simulink model "analyze"  (R2014a)
settings: Solver=FixedStepDiscrete  StartTime=0.0  StopTime=1  FixedStep=0.02  RelTol=1e-3
InitFcn:
  | Veh_Par_wxt
values from neighbouring files (symbols this model uses):
  ag_thr = 0.4*g    (= 3.924)    [Veh_Par_wxt.m]
  B = 2.25    [Veh_Par_wxt.m]
  bra_pre_em = 12    [Veh_Par_wxt.m]
  bra_pre_gz2 = 12/3    (= 4)    [Veh_Par_wxt.m]
  bra_pre_gz34 = 12/3    (= 4)    [Veh_Par_wxt.m]
  bra_pre_yd = 12/2    (= 6)    [Veh_Par_wxt.m]
  brakepre_dem_data = [0 1 2 3 4 5 6 7 8 9 10 11 12]    [Veh_Par_wxt.m]
  brakeTrq_dem_data = [0 218.198 436.396 654.594 872.792 1090.99 1309.188 1527.386 1745.584 1963.782 2181.98 2400.178 2618.376]    [Veh_Par_wxt.m]
  bratrq_max = 4*2618.376    (= 10473.504)    [Veh_Par_wxt.m]
  eff_tran = 0.75    [Veh_Par_wxt.m]
  G = Mass*g    (= 36297)    [Veh_Par_wxt.m]
  kd1 = 1    [Veh_Par_wxt.m]
  kd2 = 1    [Veh_Par_wxt.m]
  kd3 = 1    [Veh_Par_wxt.m]
  ki1 = 1    [Veh_Par_wxt.m]
  ki2 = 1    [Veh_Par_wxt.m]
  ki3 = 1    [Veh_Par_wxt.m]
  kp1 = 1    [Veh_Par_wxt.m]
  kp2 = 1    [Veh_Par_wxt.m]
  kp3 = 1    [Veh_Par_wxt.m]
  L = 3.12    [Veh_Par_wxt.m]
  premax = 12    [Veh_Par_wxt.m]
  Radius = 0.20    (= 0.2)    [Veh_Par_wxt.m]
  s_opt_yi_add = 0.05    [Veh_Par_wxt.m]
  s_opt_zhuan_add = 0.05    [Veh_Par_wxt.m]
  spd_map_mot = [0 100 200 300 360 400 500 600 700 800 900]*tras_ratio    [Veh_Par_wxt.m]
  spdmax = 900*tras_ratio    (= 5580)    [Veh_Par_wxt.m]
  speed_thr_park = 5/3.6/Radius*30/pi    (= 66.3145596216)    [Veh_Par_wxt.m]
  tras_ratio = 6.2    [Veh_Par_wxt.m]
  trq_map_mot = [1200 1200 1200 1200 1200 1080 864 720 617 540 480]/tras_ratio    [Veh_Par_wxt.m]
  trqmax = 80    [Veh_Par_wxt.m]
  v_thr1_b = 5    [Veh_Par_wxt.m]
  v_thr2_b = 20    [Veh_Par_wxt.m]
  v_thr_park = 5    [Veh_Par_wxt.m]
undefined symbols (not defined in the file or in its folder): DiscIntNeverNeededParam
libraries: simulink x231, ec5744lib x19
(part 6 of 16)

== matlab function analyze/MainControl/mode_control/backward/backward/Drive/目标转向力矩确定模块/MATLAB Function1 ==
  data: v_act input; Rturn_min_ag output; ag_thr input
function Rturn_min_ag = fcn(v_act,ag_thr)
%#codegen

    Rturn_min_ag=(v_act/3.6)^2/ag_thr;
end

== matlab function analyze/MainControl/mode_control/backward/backward/Drive/驱动防滑控制TCS/直行TCS/直行/HeartBeat1 ==
  data: life_pre input; life output
function life = fcn(life_pre)
%#codegen
life=life_pre+1;
if life>15
    life=0;
end
end

== matlab function analyze/MainControl/mode_control/backward/backward/Drive/驱动防滑控制TCS/转向TCS/MATLAB Function ==
  data: steer_dem input; y output
function y = fcn(steer_dem)
%#codegen左转为0，右转为1
if steer_dem>0
    y=0;
else
    y = 1;
end
end

== matlab function analyze/MainControl/mode_control/backward/backward/Drive/驱动防滑控制TCS/转向TCS/右转/MATLAB Function ==
  data: s_act_lf input; flag_lf output; s_opt_zhuan input; s_opt_zhuan_add input; flag_lf_pre input
function flag_lf = fcn(s_act_lf,s_opt_zhuan,s_opt_zhuan_add,flag_lf_pre)
%#codegen
if s_act_lf>s_opt_zhuan+s_opt_zhuan_add
    flag_lf=1;
elseif s_act_lf<s_opt_zhuan
    flag_lf = 0;
else
    flag_lf=flag_lf_pre;
end
end

== matlab function analyze/MainControl/mode_control/backward/backward/Drive/驱动防滑控制TCS/转向TCS/右转/前轮滑转/HeartBeat ==
  data: life_pre input; life output
function life = fcn(life_pre)
%#codegen
life=life_pre+1;
if life>15
    life=0;
end
end

== matlab function analyze/MainControl/mode_control/backward/backward/Drive/驱动防滑控制TCS/转向TCS/左转/MATLAB Function ==
  data: s_act_lf input; flag_lf output; s_opt_zhuan input; s_opt_zhuan_add input; flag_lf_pre input
function flag_lf = fcn(s_act_lf,s_opt_zhuan,s_opt_zhuan_add,flag_lf_pre)
%#codegen
if s_act_lf>s_opt_zhuan+s_opt_zhuan_add
    flag_lf=1;
elseif s_act_lf<s_opt_zhuan
    flag_lf = 0;
else
    flag_lf=flag_lf_pre;
end
end

== matlab function analyze/MainControl/mode_control/backward/backward/Drive/驱动防滑控制TCS/转向TCS/左转/前后轮均滑转/HeartBeat1 ==
  data: life_pre input; life output
function life = fcn(life_pre)
%#codegen
life=life_pre+1;
if life>15
    life=0;
end
end

== matlab function analyze/MainControl/mode_control/backward/backward/Drive/驱动防滑控制TCS/转向TCS/左转/无滑转/HeartBeat1 ==
  data: life_pre input; life output
function life = fcn(life_pre)
%#codegen
life=life_pre+1;
if life>15
    life=0;
end
end

== matlab function analyze/InputSignalProcess/MATLAB Function4 ==
  data: mode_dem input; mode_dem1 output
function mode_dem1 = fcn(mode_dem)
%#codegen
if mode_dem==0 || mode_dem==4 || mode_dem==5 
    mode_dem1=1;
elseif mode_dem==1 || mode_dem==6 || mode_dem==7 
    mode_dem1=3
elseif mode_dem==2 || mode_dem==3
    mode_dem1=4;
else 
    mode_dem1=2;
end
end

== system analyze/Data_Input/MCU1_VCU3/MCU1_VCU3 ==
  input : Inport
  Enable : EnablePort
  Demux : Demux  Outputs=8
  M2Current_Ad : Sum
  M2Current_Convert : DataTypeConversion  OutDataTypeStr=uint32
  M2Current_F : Gain  Gain=0.5
  M2Current_L : simulink/Logic and Bit Operations/Bitwise Operator  logicop=AND  UseBitMask=on  BitMask=65520  BitMaskRealWorld=Stored Integer
  M2Current_O : Constant  Value=-600  OutDataTypeStr=single
  M2Current_S : ArithShift  BitShiftNumber=4
  M2Current_Sub : Subsystem
  M2Current_sat : Saturate  UpperLimit=1447.5  LowerLimit=-600
  M2Currentcv : DataTypeConversion
  M2Currentinput3_Ad : Sum
  M2Currentinput3_C : Constant  Value=256
  M2Currentinput3_P : Product
  M2Direction_Ad : Sum
  M2Direction_Convert : DataTypeConversion  OutDataTypeStr=uint32
  M2Direction_F : Gain
  M2Direction_L : simulink/Logic and Bit Operations/Bitwise Operator  logicop=AND  UseBitMask=on  BitMask=128  BitMaskRealWorld=Stored Integer
  M2Direction_O : Constant  Value=0  OutDataTypeStr=single
  M2Direction_S : ArithShift  BitShiftNumber=7
  M2Direction_Sub : Subsystem
  M2Direction_sat : Saturate  UpperLimit=1  LowerLimit=0
  M2Directioncv : DataTypeConversion
  M2HeartBeat_Ad : Sum
  M2HeartBeat_Convert : DataTypeConversion  OutDataTypeStr=uint32
  M2HeartBeat_F : Gain
  M2HeartBeat_L : simulink/Logic and Bit Operations/Bitwise Operator  logicop=AND  UseBitMask=on  BitMask=15  BitMaskRealWorld=Stored Integer
  M2HeartBeat_O : Constant  Value=0  OutDataTypeStr=single
  M2HeartBeat_S : ArithShift
  M2HeartBeat_Sub : Subsystem
  M2HeartBeat_sat : Saturate  UpperLimit=15  LowerLimit=0
  M2HeartBeatcv : DataTypeConversion
  M2InputVolt_Ad : Sum
  M2InputVolt_Convert : DataTypeConversion  OutDataTypeStr=uint32
  M2InputVolt_F : Gain  Gain=0.25
  M2InputVolt_L : simulink/Logic and Bit Operations/Bitwise Operator  logicop=AND  UseBitMask=on  BitMask=4095  BitMaskRealWorld=Stored Integer
  M2InputVolt_O : Constant  Value=0  OutDataTypeStr=single
  M2InputVolt_S : ArithShift
  M2InputVolt_Sub : Subsystem
  M2InputVolt_sat : Saturate  UpperLimit=1023.75  LowerLimit=0
  M2InputVoltcv : DataTypeConversion
  M2InputVoltinput8_Ad : Sum
  M2InputVoltinput8_C : Constant  Value=256
  M2InputVoltinput8_P : Product
  M2Speed_Ad : Sum
  M2Speed_Convert : DataTypeConversion  OutDataTypeStr=uint32
  M2Speed_F : Gain  Gain=5
  M2Speed_L : simulink/Logic and Bit Operations/Bitwise Operator  logicop=AND  UseBitMask=on  BitMask=65535  BitMaskRealWorld=Stored Integer
  M2Speed_O : Constant  Value=-5000  OutDataTypeStr=single
  M2Speed_S : ArithShift
  M2Speed_Sub : Subsystem
  M2Speed_sat : Saturate  UpperLimit=322675  LowerLimit=-5000
  M2Speedcv : DataTypeConversion
  M2Speedinput6_Ad : Sum
  M2Speedinput6_C : Constant  Value=256
  M2Speedinput6_P : Product
  M2State_Ad : Sum
  M2State_Convert : DataTypeConversion  OutDataTypeStr=uint32
  M2State_F : Gain
  M2State_L : simulink/Logic and Bit Operations/Bitwise Operator  logicop=AND  UseBitMask=on  BitMask=112  BitMaskRealWorld=Stored Integer
  M2State_O : Constant  Value=0  OutDataTypeStr=single
  M2State_S : ArithShift  BitShiftNumber=4
  M2State_Sub : Subsystem
  M2State_sat : Saturate  UpperLimit=7  LowerLimit=0
  M2Statecv : DataTypeConversion
  M2Torque_Ad : Sum
  M2Torque_Convert : DataTypeConversion  OutDataTypeStr=uint32
  M2Torque_F : Gain  Gain=0.25
  M2Torque_L : simulink/Logic and Bit Operations/Bitwise Operator  logicop=AND  UseBitMask=on  BitMask=4095  BitMaskRealWorld=Stored Integer
  M2Torque_O : Constant  Value=-300  OutDataTypeStr=single
  M2Torque_S : ArithShift
  M2Torque_Sub : Subsystem
  M2Torque_sat : Saturate  UpperLimit=723.75  LowerLimit=-300
  M2Torquecv : DataTypeConversion
  M2Torqueinput2_Ad : Sum
  M2Torqueinput2_C : Constant  Value=256
  M2Torqueinput2_P : Product
  M2InputVolt_Out : Outport
  M2Speed_Out : Outport  Port=2
  M2Direction_Out : Outport  Port=3
  M2State_Out : Outport  Port=4
  M2HeartBeat_Out : Outport  Port=5
  M2Current_Out : Outport  Port=6
  M2Torque_Out : Outport  Port=7
  wires:
  M2Torque_F/1 -> M2Torque_Ad/1
  M2Torque_O/1 -> M2Torque_Ad/2
  M2Torque_Ad/1 -> M2Torque_sat/1
  M2Torque_sat/1 -> M2Torque_Out/1
  Demux/2 -> M2Torqueinput2_P/1, M2Currentinput3_Ad/2
  M2Torqueinput2_C/1 -> M2Torqueinput2_P/2
  M2Torqueinput2_P/1 -> M2Torqueinput2_Ad/1
  Demux/1 -> M2Torqueinput2_Ad/2
  M2Torqueinput2_Ad/1 -> M2Torque_Sub/1(In1)
  M2Torque_Sub/1(Out1) -> M2Torque_Convert/1
  M2Torque_Convert/1 -> M2Torque_L/1
  M2Torque_L/1 -> M2Torque_S/1
  M2Torque_S/1 -> M2Torquecv/1
  M2Torquecv/1 -> M2Torque_F/1
  M2State_F/1 -> M2State_Ad/1
  M2State_O/1 -> M2State_Ad/2
  M2State_Ad/1 -> M2State_sat/1
  M2State_sat/1 -> M2State_Out/1
  Demux/4 -> M2HeartBeat_Sub/1(In1), M2Direction_Sub/1(In1), M2State_Sub/1(In1)
  M2State_Sub/1(Out1) -> M2State_Convert/1
  M2State_Convert/1 -> M2State_L/1
  M2State_L/1 -> M2State_S/1
  M2State_S/1 -> M2Statecv/1
  M2Statecv/1 -> M2State_F/1
  M2Speed_F/1 -> M2Speed_Ad/1
  M2Speed_O/1 -> M2Speed_Ad/2
  M2Speed_Ad/1 -> M2Speed_sat/1
  M2Speed_sat/1 -> M2Speed_Out/1
  Demux/6 -> M2Speedinput6_P/1
  M2Speedinput6_C/1 -> M2Speedinput6_P/2
  M2Speedinput6_P/1 -> M2Speedinput6_Ad/1
  Demux/5 -> M2Speedinput6_Ad/2
  M2Speedinput6_Ad/1 -> M2Speed_Sub/1(In1)
  M2Speed_Sub/1(Out1) -> M2Speed_Convert/1
  M2Speed_Convert/1 -> M2Speed_L/1
  M2Speed_L/1 -> M2Speed_S/1
  M2Speed_S/1 -> M2Speedcv/1
  M2Speedcv/1 -> M2Speed_F/1
  M2InputVolt_F/1 -> M2InputVolt_Ad/1
  M2InputVolt_O/1 -> M2InputVolt_Ad/2
  M2InputVolt_Ad/1 -> M2InputVolt_sat/1
  M2InputVolt_sat/1 -> M2InputVolt_Out/1
  Demux/8 -> M2InputVoltinput8_P/1
  M2InputVoltinput8_C/1 -> M2InputVoltinput8_P/2
  M2InputVoltinput8_P/1 -> M2InputVoltinput8_Ad/1
  Demux/7 -> M2InputVoltinput8_Ad/2
  M2InputVoltinput8_Ad/1 -> M2InputVolt_Sub/1(In1)
  M2InputVolt_Sub/1(Out1) -> M2InputVolt_Convert/1
  M2InputVolt_Convert/1 -> M2InputVolt_L/1
  M2InputVolt_L/1 -> M2InputVolt_S/1
  M2InputVolt_S/1 -> M2InputVoltcv/1
  M2InputVoltcv/1 -> M2InputVolt_F/1
  M2HeartBeat_F/1 -> M2HeartBeat_Ad/1
  M2HeartBeat_O/1 -> M2HeartBeat_Ad/2
  M2HeartBeat_Ad/1 -> M2HeartBeat_sat/1
  M2HeartBeat_sat/1 -> M2HeartBeat_Out/1
  M2HeartBeat_Sub/1(Out1) -> M2HeartBeat_Convert/1
  M2HeartBeat_Convert/1 -> M2HeartBeat_L/1
  M2HeartBeat_L/1 -> M2HeartBeat_S/1
  M2HeartBeat_S/1 -> M2HeartBeatcv/1
  M2HeartBeatcv/1 -> M2HeartBeat_F/1
  M2Direction_F/1 -> M2Direction_Ad/1
  M2Direction_O/1 -> M2Direction_Ad/2
  M2Direction_Ad/1 -> M2Direction_sat/1
  M2Direction_sat/1 -> M2Direction_Out/1
  M2Direction_Sub/1(Out1) -> M2Direction_Convert/1
  M2Direction_Convert/1 -> M2Direction_L/1
  M2Direction_L/1 -> M2Direction_S/1
  M2Direction_S/1 -> M2Directioncv/1
  M2Directioncv/1 -> M2Direction_F/1
  M2Current_F/1 -> M2Current_Ad/1
  M2Current_O/1 -> M2Current_Ad/2
  M2Current_Ad/1 -> M2Current_sat/1
  M2Current_sat/1 -> M2Current_Out/1
  Demux/3 -> M2Currentinput3_P/1
  M2Currentinput3_C/1 -> M2Currentinput3_P/2
  M2Currentinput3_P/1 -> M2Currentinput3_Ad/1
  M2Currentinput3_Ad/1 -> M2Current_Sub/1(In1)
  M2Current_Sub/1(Out1) -> M2Current_Convert/1
  M2Current_Convert/1 -> M2Current_L/1
  M2Current_L/1 -> M2Current_S/1
  M2Current_S/1 -> M2Currentcv/1
  M2Currentcv/1 -> M2Current_F/1
  input/1 -> Demux/1

== system analyze/Data_Input/MCU1_VCU4/MCU1_VCU4 ==
  input : Inport
  Enable : EnablePort
  Demux : Demux  Outputs=8
  M2FaultCode_Ad : Sum
  M2FaultCode_Convert : DataTypeConversion  OutDataTypeStr=uint32
  M2FaultCode_F : Gain
  M2FaultCode_L : simulink/Logic and Bit Operations/Bitwise Operator  logicop=AND  UseBitMask=on  BitMask=65520  BitMaskRealWorld=Stored Integer
  M2FaultCode_O : Constant  Value=0  OutDataTypeStr=single
  M2FaultCode_S : ArithShift  BitShiftNumber=4
  M2FaultCode_Sub : Subsystem
  M2FaultCode_sat : Saturate  UpperLimit=4095  LowerLimit=0
  M2FaultCodecv : DataTypeConversion
  M2FaultCodeinput8_Ad : Sum
  M2FaultCodeinput8_C : Constant  Value=256
  M2FaultCodeinput8_P : Product
  M2FaultGrade_Ad : Sum
  M2FaultGrade_Convert : DataTypeConversion  OutDataTypeStr=uint32
  M2FaultGrade_F : Gain
  M2FaultGrade_L : simulink/Logic and Bit Operations/Bitwise Operator  logicop=AND  UseBitMask=on  BitMask=15  BitMaskRealWorld=Stored Integer
  M2FaultGrade_O : Constant  Value=0  OutDataTypeStr=single
  M2FaultGrade_S : ArithShift
  M2FaultGrade_Sub : Subsystem
  M2FaultGrade_sat : Saturate  UpperLimit=15  LowerLimit=0
  M2FaultGradecv : DataTypeConversion
  M2IGBTTemp_Ad : Sum
  M2IGBTTemp_Convert : DataTypeConversion  OutDataTypeStr=uint32
  M2IGBTTemp_F : Gain
  M2IGBTTemp_L : simulink/Logic and Bit Operations/Bitwise Operator  logicop=AND  UseBitMask=on  BitMask=255  BitMaskRealWorld=Stored Integer
  M2IGBTTemp_O : Constant  Value=-50  OutDataTypeStr=single
  M2IGBTTemp_S : ArithShift
  M2IGBTTemp_Sub : Subsystem
  M2IGBTTemp_sat : Saturate  UpperLimit=205  LowerLimit=-50
  M2IGBTTempcv : DataTypeConversion
  M2Temp_Ad : Sum
  M2Temp_Convert : DataTypeConversion  OutDataTypeStr=uint32
  M2Temp_F : Gain
  M2Temp_L : simulink/Logic and Bit Operations/Bitwise Operator  logicop=AND  UseBitMask=on  BitMask=255  BitMaskRealWorld=Stored Integer
  M2Temp_O : Constant  Value=-50  OutDataTypeStr=single
  M2Temp_S : ArithShift
  M2Temp_Sub : Subsystem
  M2Temp_sat : Saturate  UpperLimit=205  LowerLimit=-50
  M2Tempcv : DataTypeConversion
  M2TqLimit_Ad : Sum
  M2TqLimit_Convert : DataTypeConversion  OutDataTypeStr=uint32
  M2TqLimit_F : Gain  Gain=0.125
  M2TqLimit_L : simulink/Logic and Bit Operations/Bitwise Operator  logicop=AND  UseBitMask=on  BitMask=65535  BitMaskRealWorld=Stored Integer
  M2TqLimit_O : Constant  Value=0  OutDataTypeStr=single
  M2TqLimit_S : ArithShift
  M2TqLimit_Sub : Subsystem
  M2TqLimit_sat : Saturate  UpperLimit=8191.875  LowerLimit=0
  M2TqLimitcv : DataTypeConversion
  M2TqLimitinput6_Ad : Sum
  M2TqLimitinput6_C : Constant  Value=256
  M2TqLimitinput6_P : Product
  M2FaultGrade_Out : Outport
  M2FaultCode_Out : Outport  Port=2
  M2TqLimit_Out : Outport  Port=3
  M2IGBTTemp_Out : Outport  Port=4
  M2Temp_Out : Outport  Port=5
  wires:
  M2FaultCode_F/1 -> M2FaultCode_Ad/1
  M2FaultCode_O/1 -> M2FaultCode_Ad/2
  M2FaultCode_Ad/1 -> M2FaultCode_sat/1
  M2FaultCode_sat/1 -> M2FaultCode_Out/1
  Demux/8 -> M2FaultCodeinput8_P/1
  M2FaultCodeinput8_C/1 -> M2FaultCodeinput8_P/2
  M2FaultCodeinput8_P/1 -> M2FaultCodeinput8_Ad/1
  Demux/7 -> M2FaultCodeinput8_Ad/2, M2FaultGrade_Sub/1(In1)
  M2FaultCodeinput8_Ad/1 -> M2FaultCode_Sub/1(In1)
  M2FaultCode_Sub/1(Out1) -> M2FaultCode_Convert/1
  M2FaultCode_Convert/1 -> M2FaultCode_L/1
  M2FaultCode_L/1 -> M2FaultCode_S/1
  M2FaultCode_S/1 -> M2FaultCodecv/1
  M2FaultCodecv/1 -> M2FaultCode_F/1
  M2FaultGrade_F/1 -> M2FaultGrade_Ad/1
  M2FaultGrade_O/1 -> M2FaultGrade_Ad/2
  M2FaultGrade_Ad/1 -> M2FaultGrade_sat/1
  M2FaultGrade_sat/1 -> M2FaultGrade_Out/1
  M2FaultGrade_Sub/1(Out1) -> M2FaultGrade_Convert/1
  M2FaultGrade_Convert/1 -> M2FaultGrade_L/1
  M2FaultGrade_L/1 -> M2FaultGrade_S/1
  M2FaultGrade_S/1 -> M2FaultGradecv/1
  M2FaultGradecv/1 -> M2FaultGrade_F/1
  M2TqLimit_F/1 -> M2TqLimit_Ad/1
  M2TqLimit_O/1 -> M2TqLimit_Ad/2
  M2TqLimit_Ad/1 -> M2TqLimit_sat/1
  M2TqLimit_sat/1 -> M2TqLimit_Out/1
  Demux/6 -> M2TqLimitinput6_P/1
  M2TqLimitinput6_C/1 -> M2TqLimitinput6_P/2
  M2TqLimitinput6_P/1 -> M2TqLimitinput6_Ad/1
  Demux/5 -> M2TqLimitinput6_Ad/2
  M2TqLimitinput6_Ad/1 -> M2TqLimit_Sub/1(In1)
  M2TqLimit_Sub/1(Out1) -> M2TqLimit_Convert/1
  M2TqLimit_Convert/1 -> M2TqLimit_L/1
  M2TqLimit_L/1 -> M2TqLimit_S/1
  M2TqLimit_S/1 -> M2TqLimitcv/1
  M2TqLimitcv/1 -> M2TqLimit_F/1
  M2IGBTTemp_F/1 -> M2IGBTTemp_Ad/1
  M2IGBTTemp_O/1 -> M2IGBTTemp_Ad/2
  M2IGBTTemp_Ad/1 -> M2IGBTTemp_sat/1
  M2IGBTTemp_sat/1 -> M2IGBTTemp_Out/1
  Demux/2 -> M2IGBTTemp_Sub/1(In1)
  M2IGBTTemp_Sub/1(Out1) -> M2IGBTTemp_Convert/1
  M2IGBTTemp_Convert/1 -> M2IGBTTemp_L/1
  M2IGBTTemp_L/1 -> M2IGBTTemp_S/1
  M2IGBTTemp_S/1 -> M2IGBTTempcv/1
  M2IGBTTempcv/1 -> M2IGBTTemp_F/1
  M2Temp_F/1 -> M2Temp_Ad/1
  M2Temp_O/1 -> M2Temp_Ad/2
  M2Temp_Ad/1 -> M2Temp_sat/1
  M2Temp_sat/1 -> M2Temp_Out/1
  Demux/1 -> M2Temp_Sub/1(In1)
  M2Temp_Sub/1(Out1) -> M2Temp_Convert/1
  M2Temp_Convert/1 -> M2Temp_L/1
  M2Temp_L/1 -> M2Temp_S/1
  M2Temp_S/1 -> M2Tempcv/1
  M2Tempcv/1 -> M2Temp_F/1
  input/1 -> Demux/1

== system analyze/Data_Input/MCU2_VCU1/MCU2_VCU1 ==
  input : Inport
  Enable : EnablePort
  Demux : Demux  Outputs=8
  M3Current_Ad : Sum
  M3Current_Convert : DataTypeConversion  OutDataTypeStr=uint32
  M3Current_F : Gain  Gain=0.5
  M3Current_L : simulink/Logic and Bit Operations/Bitwise Operator  logicop=AND  UseBitMask=on  BitMask=65520  BitMaskRealWorld=Stored Integer
  M3Current_O : Constant  Value=-600  OutDataTypeStr=single
  M3Current_S : ArithShift  BitShiftNumber=4
  M3Current_Sub : Subsystem
  M3Current_sat : Saturate  UpperLimit=1447.5  LowerLimit=-600
  M3Currentcv : DataTypeConversion
  M3Currentinput3_Ad : Sum
  M3Currentinput3_C : Constant  Value=256
  M3Currentinput3_P : Product
  M3Direction_Ad : Sum
  M3Direction_Convert : DataTypeConversion  OutDataTypeStr=uint32
  M3Direction_F : Gain
  M3Direction_L : simulink/Logic and Bit Operations/Bitwise Operator  logicop=AND  UseBitMask=on  BitMask=128  BitMaskRealWorld=Stored Integer
  M3Direction_O : Constant  Value=0  OutDataTypeStr=single
  M3Direction_S : ArithShift  BitShiftNumber=7
  M3Direction_Sub : Subsystem
  M3Direction_sat : Saturate  UpperLimit=1  LowerLimit=0
  M3Directioncv : DataTypeConversion
  M3HeartBeat_Ad : Sum
  M3HeartBeat_Convert : DataTypeConversion  OutDataTypeStr=uint32
  M3HeartBeat_F : Gain
  M3HeartBeat_L : simulink/Logic and Bit Operations/Bitwise Operator  logicop=AND  UseBitMask=on  BitMask=15  BitMaskRealWorld=Stored Integer
  M3HeartBeat_O : Constant  Value=0  OutDataTypeStr=single
  M3HeartBeat_S : ArithShift
  M3HeartBeat_Sub : Subsystem
  M3HeartBeat_sat : Saturate  UpperLimit=15  LowerLimit=0
  M3HeartBeatcv : DataTypeConversion
  M3InputVolt_Ad : Sum
  M3InputVolt_Convert : DataTypeConversion  OutDataTypeStr=uint32
  M3InputVolt_F : Gain  Gain=0.25
  M3InputVolt_L : simulink/Logic and Bit Operations/Bitwise Operator  logicop=AND  UseBitMask=on  BitMask=4095  BitMaskRealWorld=Stored Integer
  M3InputVolt_O : Constant  Value=0  OutDataTypeStr=single
  M3InputVolt_S : ArithShift
  M3InputVolt_Sub : Subsystem
  M3InputVolt_sat : Saturate  UpperLimit=1023.75  LowerLimit=0
  M3InputVoltcv : DataTypeConversion
  M3InputVoltinput8_Ad : Sum
  M3InputVoltinput8_C : Constant  Value=256
  M3InputVoltinput8_P : Product
  M3Speed_Ad : Sum
  M3Speed_Convert : DataTypeConversion  OutDataTypeStr=uint32
  M3Speed_F : Gain  Gain=5
  M3Speed_L : simulink/Logic and Bit Operations/Bitwise Operator  logicop=AND  UseBitMask=on  BitMask=65535  BitMaskRealWorld=Stored Integer
  M3Speed_O : Constant  Value=-5000  OutDataTypeStr=single
  M3Speed_S : ArithShift
  M3Speed_Sub : Subsystem
  M3Speed_sat : Saturate  UpperLimit=322675  LowerLimit=-5000
  M3Speedcv : DataTypeConversion
  M3Speedinput6_Ad : Sum
  M3Speedinput6_C : Constant  Value=256
  M3Speedinput6_P : Product
  M3State_Ad : Sum
  M3State_Convert : DataTypeConversion  OutDataTypeStr=uint32
  M3State_F : Gain
  M3State_L : simulink/Logic and Bit Operations/Bitwise Operator  logicop=AND  UseBitMask=on  BitMask=112  BitMaskRealWorld=Stored Integer
  M3State_O : Constant  Value=0  OutDataTypeStr=single
  M3State_S : ArithShift  BitShiftNumber=4
  M3State_Sub : Subsystem
  M3State_sat : Saturate  UpperLimit=7  LowerLimit=0
  M3Statecv : DataTypeConversion
  M3Torque_Ad : Sum
  M3Torque_Convert : DataTypeConversion  OutDataTypeStr=uint32
  M3Torque_F : Gain  Gain=0.25
  M3Torque_L : simulink/Logic and Bit Operations/Bitwise Operator  logicop=AND  UseBitMask=on  BitMask=4095  BitMaskRealWorld=Stored Integer
  M3Torque_O : Constant  Value=-300  OutDataTypeStr=single
  M3Torque_S : ArithShift
  M3Torque_Sub : Subsystem
  M3Torque_sat : Saturate  UpperLimit=723.75  LowerLimit=-300
  M3Torquecv : DataTypeConversion
  M3Torqueinput2_Ad : Sum
  M3Torqueinput2_C : Constant  Value=256
  M3Torqueinput2_P : Product
  M3InputVolt_Out : Outport
  M3Speed_Out : Outport  Port=2
  M3Direction_Out : Outport  Port=3
  M3State_Out : Outport  Port=4
  M3HeartBeat_Out : Outport  Port=5
  M3Current_Out : Outport  Port=6
  M3Torque_Out : Outport  Port=7
  wires:
  M3InputVolt_F/1 -> M3InputVolt_Ad/1
  M3InputVolt_O/1 -> M3InputVolt_Ad/2
  M3InputVolt_Ad/1 -> M3InputVolt_sat/1
  M3InputVolt_sat/1 -> M3InputVolt_Out/1
  Demux/8 -> M3InputVoltinput8_P/1
  M3InputVoltinput8_C/1 -> M3InputVoltinput8_P/2
  M3InputVoltinput8_P/1 -> M3InputVoltinput8_Ad/1
  Demux/7 -> M3InputVoltinput8_Ad/2
  M3InputVoltinput8_Ad/1 -> M3InputVolt_Sub/1(In1)
  M3InputVolt_Sub/1(Out1) -> M3InputVolt_Convert/1
  M3InputVolt_Convert/1 -> M3InputVolt_L/1
  M3InputVolt_L/1 -> M3InputVolt_S/1
  M3InputVolt_S/1 -> M3InputVoltcv/1
  M3InputVoltcv/1 -> M3InputVolt_F/1
  M3Speed_F/1 -> M3Speed_Ad/1
  M3Speed_O/1 -> M3Speed_Ad/2
  M3Speed_Ad/1 -> M3Speed_sat/1
  M3Speed_sat/1 -> M3Speed_Out/1
  Demux/6 -> M3Speedinput6_P/1
  M3Speedinput6_C/1 -> M3Speedinput6_P/2
  M3Speedinput6_P/1 -> M3Speedinput6_Ad/1
  Demux/5 -> M3Speedinput6_Ad/2
  M3Speedinput6_Ad/1 -> M3Speed_Sub/1(In1)
  M3Speed_Sub/1(Out1) -> M3Speed_Convert/1
  M3Speed_Convert/1 -> M3Speed_L/1
  M3Speed_L/1 -> M3Speed_S/1
  M3Speed_S/1 -> M3Speedcv/1
  M3Speedcv/1 -> M3Speed_F/1
  M3Direction_F/1 -> M3Direction_Ad/1
  M3Direction_O/1 -> M3Direction_Ad/2
  M3Direction_Ad/1 -> M3Direction_sat/1
  M3Direction_sat/1 -> M3Direction_Out/1
  Demux/4 -> M3State_Sub/1(In1), M3HeartBeat_Sub/1(In1), M3Direction_Sub/1(In1)
  M3Direction_Sub/1(Out1) -> M3Direction_Convert/1
  M3Direction_Convert/1 -> M3Direction_L/1
  M3Direction_L/1 -> M3Direction_S/1
  M3Direction_S/1 -> M3Directioncv/1
  M3Directioncv/1 -> M3Direction_F/1
  M3State_F/1 -> M3State_Ad/1
  M3State_O/1 -> M3State_Ad/2
  M3State_Ad/1 -> M3State_sat/1
  M3State_sat/1 -> M3State_Out/1
  M3State_Sub/1(Out1) -> M3State_Convert/1
  M3State_Convert/1 -> M3State_L/1
  M3State_L/1 -> M3State_S/1
  M3State_S/1 -> M3Statecv/1
  M3Statecv/1 -> M3State_F/1
  M3HeartBeat_F/1 -> M3HeartBeat_Ad/1
  M3HeartBeat_O/1 -> M3HeartBeat_Ad/2
  M3HeartBeat_Ad/1 -> M3HeartBeat_sat/1
  M3HeartBeat_sat/1 -> M3HeartBeat_Out/1
  M3HeartBeat_Sub/1(Out1) -> M3HeartBeat_Convert/1
  M3HeartBeat_Convert/1 -> M3HeartBeat_L/1
  M3HeartBeat_L/1 -> M3HeartBeat_S/1
  M3HeartBeat_S/1 -> M3HeartBeatcv/1
  M3HeartBeatcv/1 -> M3HeartBeat_F/1
  M3Current_F/1 -> M3Current_Ad/1
  M3Current_O/1 -> M3Current_Ad/2
  M3Current_Ad/1 -> M3Current_sat/1
  M3Current_sat/1 -> M3Current_Out/1
  Demux/3 -> M3Currentinput3_P/1
  M3Currentinput3_C/1 -> M3Currentinput3_P/2
  M3Currentinput3_P/1 -> M3Currentinput3_Ad/1
  Demux/2 -> M3Currentinput3_Ad/2, M3Torqueinput2_P/1
  M3Currentinput3_Ad/1 -> M3Current_Sub/1(In1)
  M3Current_Sub/1(Out1) -> M3Current_Convert/1
  M3Current_Convert/1 -> M3Current_L/1
  M3Current_L/1 -> M3Current_S/1
  M3Current_S/1 -> M3Currentcv/1
  M3Currentcv/1 -> M3Current_F/1
  M3Torque_F/1 -> M3Torque_Ad/1
  M3Torque_O/1 -> M3Torque_Ad/2
  M3Torque_Ad/1 -> M3Torque_sat/1
  M3Torque_sat/1 -> M3Torque_Out/1
  M3Torqueinput2_C/1 -> M3Torqueinput2_P/2
  M3Torqueinput2_P/1 -> M3Torqueinput2_Ad/1
  Demux/1 -> M3Torqueinput2_Ad/2
  M3Torqueinput2_Ad/1 -> M3Torque_Sub/1(In1)
  M3Torque_Sub/1(Out1) -> M3Torque_Convert/1
  M3Torque_Convert/1 -> M3Torque_L/1
  M3Torque_L/1 -> M3Torque_S/1
  M3Torque_S/1 -> M3Torquecv/1
  M3Torquecv/1 -> M3Torque_F/1
  input/1 -> Demux/1

== system analyze/Data_Input/MCU2_VCU2/MCU2_VCU2 ==
  input : Inport
  Enable : EnablePort
  Demux : Demux  Outputs=8
  M3FaultCode_Ad : Sum
  M3FaultCode_Convert : DataTypeConversion  OutDataTypeStr=uint32
  M3FaultCode_F : Gain
  M3FaultCode_L : simulink/Logic and Bit Operations/Bitwise Operator  logicop=AND  UseBitMask=on  BitMask=65520  BitMaskRealWorld=Stored Integer
  M3FaultCode_O : Constant  Value=0  OutDataTypeStr=single
  M3FaultCode_S : ArithShift  BitShiftNumber=4
  M3FaultCode_Sub : Subsystem
  M3FaultCode_sat : Saturate  UpperLimit=4095  LowerLimit=0
  M3FaultCodecv : DataTypeConversion
  M3FaultCodeinput8_Ad : Sum
  M3FaultCodeinput8_C : Constant  Value=256
  M3FaultCodeinput8_P : Product
  M3FaultGrade_Ad : Sum
  M3FaultGrade_Convert : DataTypeConversion  OutDataTypeStr=uint32
  M3FaultGrade_F : Gain
  M3FaultGrade_L : simulink/Logic and Bit Operations/Bitwise Operator  logicop=AND  UseBitMask=on  BitMask=15  BitMaskRealWorld=Stored Integer
  M3FaultGrade_O : Constant  Value=0  OutDataTypeStr=single
  M3FaultGrade_S : ArithShift
  M3FaultGrade_Sub : Subsystem
  M3FaultGrade_sat : Saturate  UpperLimit=15  LowerLimit=0
  M3FaultGradecv : DataTypeConversion
  M3IGBTTemp_Ad : Sum
  M3IGBTTemp_Convert : DataTypeConversion  OutDataTypeStr=uint32
  M3IGBTTemp_F : Gain
  M3IGBTTemp_L : simulink/Logic and Bit Operations/Bitwise Operator  logicop=AND  UseBitMask=on  BitMask=255  BitMaskRealWorld=Stored Integer
  M3IGBTTemp_O : Constant  Value=-50  OutDataTypeStr=single
  M3IGBTTemp_S : ArithShift
  M3IGBTTemp_Sub : Subsystem
  M3IGBTTemp_sat : Saturate  UpperLimit=205  LowerLimit=-50
  M3IGBTTempcv : DataTypeConversion
  M3Temp_Ad : Sum
  M3Temp_Convert : DataTypeConversion  OutDataTypeStr=uint32
  M3Temp_F : Gain
  M3Temp_L : simulink/Logic and Bit Operations/Bitwise Operator  logicop=AND  UseBitMask=on  BitMask=255  BitMaskRealWorld=Stored Integer
  M3Temp_O : Constant  Value=-50  OutDataTypeStr=single
  M3Temp_S : ArithShift
  M3Temp_Sub : Subsystem
  M3Temp_sat : Saturate  UpperLimit=205  LowerLimit=-50
  M3Tempcv : DataTypeConversion
  M3TqLimit_Ad : Sum
  M3TqLimit_Convert : DataTypeConversion  OutDataTypeStr=uint32
  M3TqLimit_F : Gain  Gain=0.125
  M3TqLimit_L : simulink/Logic and Bit Operations/Bitwise Operator  logicop=AND  UseBitMask=on  BitMask=65535  BitMaskRealWorld=Stored Integer
  M3TqLimit_O : Constant  Value=0  OutDataTypeStr=single
  M3TqLimit_S : ArithShift
  M3TqLimit_Sub : Subsystem
  M3TqLimit_sat : Saturate  UpperLimit=8191.875  LowerLimit=0
  M3TqLimitcv : DataTypeConversion
  M3TqLimitinput6_Ad : Sum
  M3TqLimitinput6_C : Constant  Value=256
  M3TqLimitinput6_P : Product
  M3FaultGrade_Out : Outport
  M3FaultCode_Out : Outport  Port=2
  M3TqLimit_Out : Outport  Port=3
  M3IGBTTemp_Out : Outport  Port=4
  M3Temp_Out : Outport  Port=5
  wires:
  M3FaultCode_F/1 -> M3FaultCode_Ad/1
  M3FaultCode_O/1 -> M3FaultCode_Ad/2
  M3FaultCode_Ad/1 -> M3FaultCode_sat/1
  M3FaultCode_sat/1 -> M3FaultCode_Out/1
  Demux/8 -> M3FaultCodeinput8_P/1
  M3FaultCodeinput8_C/1 -> M3FaultCodeinput8_P/2
  M3FaultCodeinput8_P/1 -> M3FaultCodeinput8_Ad/1
  Demux/7 -> M3FaultCodeinput8_Ad/2, M3FaultGrade_Sub/1(In1)
  M3FaultCodeinput8_Ad/1 -> M3FaultCode_Sub/1(In1)
  M3FaultCode_Sub/1(Out1) -> M3FaultCode_Convert/1
  M3FaultCode_Convert/1 -> M3FaultCode_L/1
  M3FaultCode_L/1 -> M3FaultCode_S/1
  M3FaultCode_S/1 -> M3FaultCodecv/1
  M3FaultCodecv/1 -> M3FaultCode_F/1
  M3FaultGrade_F/1 -> M3FaultGrade_Ad/1
  M3FaultGrade_O/1 -> M3FaultGrade_Ad/2
  M3FaultGrade_Ad/1 -> M3FaultGrade_sat/1
  M3FaultGrade_sat/1 -> M3FaultGrade_Out/1
  M3FaultGrade_Sub/1(Out1) -> M3FaultGrade_Convert/1
  M3FaultGrade_Convert/1 -> M3FaultGrade_L/1
  M3FaultGrade_L/1 -> M3FaultGrade_S/1
  M3FaultGrade_S/1 -> M3FaultGradecv/1
  M3FaultGradecv/1 -> M3FaultGrade_F/1
  M3TqLimit_F/1 -> M3TqLimit_Ad/1
  M3TqLimit_O/1 -> M3TqLimit_Ad/2
  M3TqLimit_Ad/1 -> M3TqLimit_sat/1
  M3TqLimit_sat/1 -> M3TqLimit_Out/1
  Demux/6 -> M3TqLimitinput6_P/1
  M3TqLimitinput6_C/1 -> M3TqLimitinput6_P/2
  M3TqLimitinput6_P/1 -> M3TqLimitinput6_Ad/1
  Demux/5 -> M3TqLimitinput6_Ad/2
  M3TqLimitinput6_Ad/1 -> M3TqLimit_Sub/1(In1)
  M3TqLimit_Sub/1(Out1) -> M3TqLimit_Convert/1
  M3TqLimit_Convert/1 -> M3TqLimit_L/1
  M3TqLimit_L/1 -> M3TqLimit_S/1
  M3TqLimit_S/1 -> M3TqLimitcv/1
  M3TqLimitcv/1 -> M3TqLimit_F/1
  M3IGBTTemp_F/1 -> M3IGBTTemp_Ad/1
  M3IGBTTemp_O/1 -> M3IGBTTemp_Ad/2
  M3IGBTTemp_Ad/1 -> M3IGBTTemp_sat/1
  M3IGBTTemp_sat/1 -> M3IGBTTemp_Out/1
  Demux/2 -> M3IGBTTemp_Sub/1(In1)
  M3IGBTTemp_Sub/1(Out1) -> M3IGBTTemp_Convert/1
  M3IGBTTemp_Convert/1 -> M3IGBTTemp_L/1
  M3IGBTTemp_L/1 -> M3IGBTTemp_S/1
  M3IGBTTemp_S/1 -> M3IGBTTempcv/1
  M3IGBTTempcv/1 -> M3IGBTTemp_F/1
  M3Temp_F/1 -> M3Temp_Ad/1
  M3Temp_O/1 -> M3Temp_Ad/2
  M3Temp_Ad/1 -> M3Temp_sat/1
  M3Temp_sat/1 -> M3Temp_Out/1
  Demux/1 -> M3Temp_Sub/1(In1)
  M3Temp_Sub/1(Out1) -> M3Temp_Convert/1
  M3Temp_Convert/1 -> M3Temp_L/1
  M3Temp_L/1 -> M3Temp_S/1
  M3Temp_S/1 -> M3Tempcv/1
  M3Tempcv/1 -> M3Temp_F/1
  input/1 -> Demux/1

== system analyze/Data_Input/MCU2_VCU3/MCU2_VCU3 ==
  input : Inport
  Enable : EnablePort
  Demux : Demux  Outputs=8
  M4Current_Ad : Sum
  M4Current_Convert : DataTypeConversion  OutDataTypeStr=uint32
  M4Current_F : Gain  Gain=0.5
  M4Current_L : simulink/Logic and Bit Operations/Bitwise Operator  logicop=AND  UseBitMask=on  BitMask=65520  BitMaskRealWorld=Stored Integer
  M4Current_O : Constant  Value=-600  OutDataTypeStr=single
  M4Current_S : ArithShift  BitShiftNumber=4
  M4Current_Sub : Subsystem
  M4Current_sat : Saturate  UpperLimit=1447.5  LowerLimit=-600
  M4Currentcv : DataTypeConversion
  M4Currentinput3_Ad : Sum
  M4Currentinput3_C : Constant  Value=256
  M4Currentinput3_P : Product
  M4Direction_Ad : Sum
  M4Direction_Convert : DataTypeConversion  OutDataTypeStr=uint32
  M4Direction_F : Gain
  M4Direction_L : simulink/Logic and Bit Operations/Bitwise Operator  logicop=AND  UseBitMask=on  BitMask=128  BitMaskRealWorld=Stored Integer
  M4Direction_O : Constant  Value=0  OutDataTypeStr=single
  M4Direction_S : ArithShift  BitShiftNumber=7
  M4Direction_Sub : Subsystem
  M4Direction_sat : Saturate  UpperLimit=1  LowerLimit=0
  M4Directioncv : DataTypeConversion
  M4HeartBeat_Ad : Sum
  M4HeartBeat_Convert : DataTypeConversion  OutDataTypeStr=uint32
  M4HeartBeat_F : Gain
  M4HeartBeat_L : simulink/Logic and Bit Operations/Bitwise Operator  logicop=AND  UseBitMask=on  BitMask=15  BitMaskRealWorld=Stored Integer
  M4HeartBeat_O : Constant  Value=0  OutDataTypeStr=single
  M4HeartBeat_S : ArithShift
  M4HeartBeat_Sub : Subsystem
  M4HeartBeat_sat : Saturate  UpperLimit=15  LowerLimit=0
  M4HeartBeatcv : DataTypeConversion
  M4InputVolt_Ad : Sum
  M4InputVolt_Convert : DataTypeConversion  OutDataTypeStr=uint32
  M4InputVolt_F : Gain  Gain=0.25
  M4InputVolt_L : simulink/Logic and Bit Operations/Bitwise Operator  logicop=AND  UseBitMask=on  BitMask=4095  BitMaskRealWorld=Stored Integer
  M4InputVolt_O : Constant  Value=0  OutDataTypeStr=single
  M4InputVolt_S : ArithShift
  M4InputVolt_Sub : Subsystem
  M4InputVolt_sat : Saturate  UpperLimit=1023.75  LowerLimit=0
  M4InputVoltcv : DataTypeConversion
  M4InputVoltinput8_Ad : Sum
  M4InputVoltinput8_C : Constant  Value=256
  M4InputVoltinput8_P : Product
  M4Speed_Ad : Sum
  M4Speed_Convert : DataTypeConversion  OutDataTypeStr=uint32
  M4Speed_F : Gain  Gain=5
  M4Speed_L : simulink/Logic and Bit Operations/Bitwise Operator  logicop=AND  UseBitMask=on  BitMask=65535  BitMaskRealWorld=Stored Integer
  M4Speed_O : Constant  Value=-5000  OutDataTypeStr=single
  M4Speed_S : ArithShift
  M4Speed_Sub : Subsystem
  M4Speed_sat : Saturate  UpperLimit=322675  LowerLimit=-5000
  M4Speedcv : DataTypeConversion
  M4Speedinput6_Ad : Sum
  M4Speedinput6_C : Constant  Value=256
  M4Speedinput6_P : Product
  M4State_Ad : Sum
  M4State_Convert : DataTypeConversion  OutDataTypeStr=uint32
  M4State_F : Gain
  M4State_L : simulink/Logic and Bit Operations/Bitwise Operator  logicop=AND  UseBitMask=on  BitMask=112  BitMaskRealWorld=Stored Integer
  M4State_O : Constant  Value=0  OutDataTypeStr=single
  M4State_S : ArithShift  BitShiftNumber=4
  M4State_Sub : Subsystem
  M4State_sat : Saturate  UpperLimit=7  LowerLimit=0
  M4Statecv : DataTypeConversion
  M4Torque_Ad : Sum
  M4Torque_Convert : DataTypeConversion  OutDataTypeStr=uint32
  M4Torque_F : Gain  Gain=0.25
  M4Torque_L : simulink/Logic and Bit Operations/Bitwise Operator  logicop=AND  UseBitMask=on  BitMask=4095  BitMaskRealWorld=Stored Integer
  M4Torque_O : Constant  Value=-300  OutDataTypeStr=single
  M4Torque_S : ArithShift
  M4Torque_Sub : Subsystem
  M4Torque_sat : Saturate  UpperLimit=723.75  LowerLimit=-300
  M4Torquecv : DataTypeConversion
  M4Torqueinput2_Ad : Sum
  M4Torqueinput2_C : Constant  Value=256
  M4Torqueinput2_P : Product
  M4InputVolt_Out : Outport
  M4Speed_Out : Outport  Port=2
  M4Direction_Out : Outport  Port=3
  M4State_Out : Outport  Port=4
  M4HeartBeat_Out : Outport  Port=5
  M4Current_Out : Outport  Port=6
  M4Torque_Out : Outport  Port=7
  wires:
  M4InputVolt_F/1 -> M4InputVolt_Ad/1
  M4InputVolt_O/1 -> M4InputVolt_Ad/2
  M4InputVolt_Ad/1 -> M4InputVolt_sat/1
  M4InputVolt_sat/1 -> M4InputVolt_Out/1
  Demux/8 -> M4InputVoltinput8_P/1
  M4InputVoltinput8_C/1 -> M4InputVoltinput8_P/2
  M4InputVoltinput8_P/1 -> M4InputVoltinput8_Ad/1
  Demux/7 -> M4InputVoltinput8_Ad/2
  M4InputVoltinput8_Ad/1 -> M4InputVolt_Sub/1(In1)
  M4InputVolt_Sub/1(Out1) -> M4InputVolt_Convert/1
  M4InputVolt_Convert/1 -> M4InputVolt_L/1
  M4InputVolt_L/1 -> M4InputVolt_S/1
  M4InputVolt_S/1 -> M4InputVoltcv/1
  M4InputVoltcv/1 -> M4InputVolt_F/1
  M4Speed_F/1 -> M4Speed_Ad/1
  M4Speed_O/1 -> M4Speed_Ad/2
  M4Speed_Ad/1 -> M4Speed_sat/1
  M4Speed_sat/1 -> M4Speed_Out/1
  Demux/6 -> M4Speedinput6_P/1
  M4Speedinput6_C/1 -> M4Speedinput6_P/2
  M4Speedinput6_P/1 -> M4Speedinput6_Ad/1
  Demux/5 -> M4Speedinput6_Ad/2
  M4Speedinput6_Ad/1 -> M4Speed_Sub/1(In1)
  M4Speed_Sub/1(Out1) -> M4Speed_Convert/1
  M4Speed_Convert/1 -> M4Speed_L/1
  M4Speed_L/1 -> M4Speed_S/1
  M4Speed_S/1 -> M4Speedcv/1
  M4Speedcv/1 -> M4Speed_F/1
  M4Direction_F/1 -> M4Direction_Ad/1
  M4Direction_O/1 -> M4Direction_Ad/2
  M4Direction_Ad/1 -> M4Direction_sat/1
  M4Direction_sat/1 -> M4Direction_Out/1
  Demux/4 -> M4State_Sub/1(In1), M4HeartBeat_Sub/1(In1), M4Direction_Sub/1(In1)
  M4Direction_Sub/1(Out1) -> M4Direction_Convert/1
  M4Direction_Convert/1 -> M4Direction_L/1
  M4Direction_L/1 -> M4Direction_S/1
  M4Direction_S/1 -> M4Directioncv/1
  M4Directioncv/1 -> M4Direction_F/1
  M4State_F/1 -> M4State_Ad/1
  M4State_O/1 -> M4State_Ad/2
  M4State_Ad/1 -> M4State_sat/1
  M4State_sat/1 -> M4State_Out/1
  M4State_Sub/1(Out1) -> M4State_Convert/1
  M4State_Convert/1 -> M4State_L/1
  M4State_L/1 -> M4State_S/1
  M4State_S/1 -> M4Statecv/1
  M4Statecv/1 -> M4State_F/1
  M4HeartBeat_F/1 -> M4HeartBeat_Ad/1
  M4HeartBeat_O/1 -> M4HeartBeat_Ad/2
  M4HeartBeat_Ad/1 -> M4HeartBeat_sat/1
  M4HeartBeat_sat/1 -> M4HeartBeat_Out/1
  M4HeartBeat_Sub/1(Out1) -> M4HeartBeat_Convert/1
  M4HeartBeat_Convert/1 -> M4HeartBeat_L/1
  M4HeartBeat_L/1 -> M4HeartBeat_S/1
  M4HeartBeat_S/1 -> M4HeartBeatcv/1
  M4HeartBeatcv/1 -> M4HeartBeat_F/1
  M4Current_F/1 -> M4Current_Ad/1
  M4Current_O/1 -> M4Current_Ad/2
  M4Current_Ad/1 -> M4Current_sat/1
  M4Current_sat/1 -> M4Current_Out/1
  Demux/3 -> M4Currentinput3_P/1
  M4Currentinput3_C/1 -> M4Currentinput3_P/2
  M4Currentinput3_P/1 -> M4Currentinput3_Ad/1
  Demux/2 -> M4Currentinput3_Ad/2, M4Torqueinput2_P/1
  M4Currentinput3_Ad/1 -> M4Current_Sub/1(In1)
  M4Current_Sub/1(Out1) -> M4Current_Convert/1
  M4Current_Convert/1 -> M4Current_L/1
  M4Current_L/1 -> M4Current_S/1
  M4Current_S/1 -> M4Currentcv/1
  M4Currentcv/1 -> M4Current_F/1
  M4Torque_F/1 -> M4Torque_Ad/1
  M4Torque_O/1 -> M4Torque_Ad/2
  M4Torque_Ad/1 -> M4Torque_sat/1
  M4Torque_sat/1 -> M4Torque_Out/1
  M4Torqueinput2_C/1 -> M4Torqueinput2_P/2
  M4Torqueinput2_P/1 -> M4Torqueinput2_Ad/1
  Demux/1 -> M4Torqueinput2_Ad/2
  M4Torqueinput2_Ad/1 -> M4Torque_Sub/1(In1)
  M4Torque_Sub/1(Out1) -> M4Torque_Convert/1
  M4Torque_Convert/1 -> M4Torque_L/1
  M4Torque_L/1 -> M4Torque_S/1
  M4Torque_S/1 -> M4Torquecv/1
  M4Torquecv/1 -> M4Torque_F/1
  input/1 -> Demux/1

== system analyze/Data_Input/MCU2_VCU4/MCU2_VCU4 ==
  input : Inport
  Enable : EnablePort
  Demux : Demux  Outputs=8
  M4FaultCode_Ad : Sum
  M4FaultCode_Convert : DataTypeConversion  OutDataTypeStr=uint32
  M4FaultCode_F : Gain
  M4FaultCode_L : simulink/Logic and Bit Operations/Bitwise Operator  logicop=AND  UseBitMask=on  BitMask=65520  BitMaskRealWorld=Stored Integer
  M4FaultCode_O : Constant  Value=0  OutDataTypeStr=single
  M4FaultCode_S : ArithShift  BitShiftNumber=4
  M4FaultCode_Sub : Subsystem
  M4FaultCode_sat : Saturate  UpperLimit=4095  LowerLimit=0
  M4FaultCodecv : DataTypeConversion
  M4FaultCodeinput8_Ad : Sum
  M4FaultCodeinput8_C : Constant  Value=256
  M4FaultCodeinput8_P : Product
  M4FaultGrade_Ad : Sum
  M4FaultGrade_Convert : DataTypeConversion  OutDataTypeStr=uint32
  M4FaultGrade_F : Gain
  M4FaultGrade_L : simulink/Logic and Bit Operations/Bitwise Operator  logicop=AND  UseBitMask=on  BitMask=15  BitMaskRealWorld=Stored Integer
  M4FaultGrade_O : Constant  Value=0  OutDataTypeStr=single
  M4FaultGrade_S : ArithShift
  M4FaultGrade_Sub : Subsystem
  M4FaultGrade_sat : Saturate  UpperLimit=15  LowerLimit=0
  M4FaultGradecv : DataTypeConversion
  M4IGBTTemp_Ad : Sum
  M4IGBTTemp_Convert : DataTypeConversion  OutDataTypeStr=uint32
  M4IGBTTemp_F : Gain
  M4IGBTTemp_L : simulink/Logic and Bit Operations/Bitwise Operator  logicop=AND  UseBitMask=on  BitMask=255  BitMaskRealWorld=Stored Integer
  M4IGBTTemp_O : Constant  Value=-50  OutDataTypeStr=single
  M4IGBTTemp_S : ArithShift
  M4IGBTTemp_Sub : Subsystem
  M4IGBTTemp_sat : Saturate  UpperLimit=205  LowerLimit=-50
  M4IGBTTempcv : DataTypeConversion
  M4Temp_Ad : Sum
  M4Temp_Convert : DataTypeConversion  OutDataTypeStr=uint32
  M4Temp_F : Gain
  M4Temp_L : simulink/Logic and Bit Operations/Bitwise Operator  logicop=AND  UseBitMask=on  BitMask=255  BitMaskRealWorld=Stored Integer
  M4Temp_O : Constant  Value=-50  OutDataTypeStr=single
  M4Temp_S : ArithShift
  M4Temp_Sub : Subsystem
  M4Temp_sat : Saturate  UpperLimit=205  LowerLimit=-50
  M4Tempcv : DataTypeConversion
  M4TqLimit_Ad : Sum
  M4TqLimit_Convert : DataTypeConversion  OutDataTypeStr=uint32
  M4TqLimit_F : Gain  Gain=0.125
  M4TqLimit_L : simulink/Logic and Bit Operations/Bitwise Operator  logicop=AND  UseBitMask=on  BitMask=65535  BitMaskRealWorld=Stored Integer
  M4TqLimit_O : Constant  Value=0  OutDataTypeStr=single
  M4TqLimit_S : ArithShift
  M4TqLimit_Sub : Subsystem
  M4TqLimit_sat : Saturate  UpperLimit=8191.875  LowerLimit=0
  M4TqLimitcv : DataTypeConversion
  M4TqLimitinput6_Ad : Sum
  M4TqLimitinput6_C : Constant  Value=256
  M4TqLimitinput6_P : Product
  M4FaultGrade_Out : Outport
  M4FaultCode_Out : Outport  Port=2
  M4TqLimit_Out : Outport  Port=3
  M4IGBTTemp_Out : Outport  Port=4
  M4Temp_Out : Outport  Port=5
  wires:
  M4FaultCode_F/1 -> M4FaultCode_Ad/1
  M4FaultCode_O/1 -> M4FaultCode_Ad/2
  M4FaultCode_Ad/1 -> M4FaultCode_sat/1
  M4FaultCode_sat/1 -> M4FaultCode_Out/1
  Demux/8 -> M4FaultCodeinput8_P/1
  M4FaultCodeinput8_C/1 -> M4FaultCodeinput8_P/2
  M4FaultCodeinput8_P/1 -> M4FaultCodeinput8_Ad/1
  Demux/7 -> M4FaultCodeinput8_Ad/2, M4FaultGrade_Sub/1(In1)
  M4FaultCodeinput8_Ad/1 -> M4FaultCode_Sub/1(In1)
  M4FaultCode_Sub/1(Out1) -> M4FaultCode_Convert/1
  M4FaultCode_Convert/1 -> M4FaultCode_L/1
  M4FaultCode_L/1 -> M4FaultCode_S/1
  M4FaultCode_S/1 -> M4FaultCodecv/1
  M4FaultCodecv/1 -> M4FaultCode_F/1
  M4FaultGrade_F/1 -> M4FaultGrade_Ad/1
  M4FaultGrade_O/1 -> M4FaultGrade_Ad/2
  M4FaultGrade_Ad/1 -> M4FaultGrade_sat/1
  M4FaultGrade_sat/1 -> M4FaultGrade_Out/1
  M4FaultGrade_Sub/1(Out1) -> M4FaultGrade_Convert/1
  M4FaultGrade_Convert/1 -> M4FaultGrade_L/1
  M4FaultGrade_L/1 -> M4FaultGrade_S/1
  M4FaultGrade_S/1 -> M4FaultGradecv/1
  M4FaultGradecv/1 -> M4FaultGrade_F/1
  M4TqLimit_F/1 -> M4TqLimit_Ad/1
  M4TqLimit_O/1 -> M4TqLimit_Ad/2
  M4TqLimit_Ad/1 -> M4TqLimit_sat/1
  M4TqLimit_sat/1 -> M4TqLimit_Out/1
  Demux/6 -> M4TqLimitinput6_P/1
  M4TqLimitinput6_C/1 -> M4TqLimitinput6_P/2
  M4TqLimitinput6_P/1 -> M4TqLimitinput6_Ad/1
  Demux/5 -> M4TqLimitinput6_Ad/2
  M4TqLimitinput6_Ad/1 -> M4TqLimit_Sub/1(In1)
  M4TqLimit_Sub/1(Out1) -> M4TqLimit_Convert/1
  M4TqLimit_Convert/1 -> M4TqLimit_L/1
  M4TqLimit_L/1 -> M4TqLimit_S/1
  M4TqLimit_S/1 -> M4TqLimitcv/1
  M4TqLimitcv/1 -> M4TqLimit_F/1
  M4IGBTTemp_F/1 -> M4IGBTTemp_Ad/1
  M4IGBTTemp_O/1 -> M4IGBTTemp_Ad/2
  M4IGBTTemp_Ad/1 -> M4IGBTTemp_sat/1
  M4IGBTTemp_sat/1 -> M4IGBTTemp_Out/1
  Demux/2 -> M4IGBTTemp_Sub/1(In1)
  M4IGBTTemp_Sub/1(Out1) -> M4IGBTTemp_Convert/1
  M4IGBTTemp_Convert/1 -> M4IGBTTemp_L/1
  M4IGBTTemp_L/1 -> M4IGBTTemp_S/1
  M4IGBTTemp_S/1 -> M4IGBTTempcv/1
  M4IGBTTempcv/1 -> M4IGBTTemp_F/1
  M4Temp_F/1 -> M4Temp_Ad/1
  M4Temp_O/1 -> M4Temp_Ad/2
  M4Temp_Ad/1 -> M4Temp_sat/1
  M4Temp_sat/1 -> M4Temp_Out/1
  Demux/1 -> M4Temp_Sub/1(In1)
  M4Temp_Sub/1(Out1) -> M4Temp_Convert/1
  M4Temp_Convert/1 -> M4Temp_L/1
  M4Temp_L/1 -> M4Temp_S/1
  M4Temp_S/1 -> M4Tempcv/1
  M4Tempcv/1 -> M4Temp_F/1
  input/1 -> Demux/1

== system analyze/MainControl/mode_control/Park ==
  Signals : Inport
  Action Port : ActionPort  ActionType=case
  Mux : Mux  Inputs=6
  park : Subsystem
  park_dem : Outport
  wires:
  Signals/1 -> park/1(Signals)
  park/4(mot_rr) -> Mux/4
  park/3(mot_rf) -> Mux/3
  park/5(bra_pre_l) -> Mux/5
  park/2(mot_lr) -> Mux/2
  park/6(bra_pre_r) -> Mux/6
  park/1(mot_lf) -> Mux/1
  Mux/1 -> park_dem/1

== system analyze/MainControl/mode_control/backward ==
  Signals : Inport
  Action Port : ActionPort  ActionType=case
  backward : Subsystem
  backward_dem : Outport
  wires:
  Signals/1 -> backward/1(Signals)
  backward/1(backward_dem) -> backward_dem/1

== system analyze/MainControl/mode_control/center_steer ==
  Signals : Inport
  Action Port : ActionPort  ActionType=case
  Mux : Mux  Inputs=6
  center_steer : Subsystem
  center_steer_dem : Outport
  wires:
  Mux/1 -> center_steer_dem/1
  center_steer/6(bra_pre_r) -> Mux/6
  center_steer/5(bra_pre_l) -> Mux/5
  Signals/1 -> center_steer/1(Signals)
  center_steer/1(mot_lf) -> Mux/1
  center_steer/2(mot_lr) -> Mux/2
  center_steer/4(mot_rr) -> Mux/4
  center_steer/3(mot_rf) -> Mux/3

== system analyze/MainControl/mode_control/emergency_stop ==
  Signals : Inport
  Action Port : ActionPort  ActionType=case
  Mux : Mux  Inputs=6
  emergency_stop : Subsystem
  emergency_stop_dem : Outport
  wires:
  Mux/1 -> emergency_stop_dem/1
  emergency_stop/1(mot_lf) -> Mux/1
  emergency_stop/6(bra_pre_r) -> Mux/6
  emergency_stop/4(mot_rr) -> Mux/4
  emergency_stop/5(bra_pre_l) -> Mux/5
  emergency_stop/3(mot_rf) -> Mux/3
  emergency_stop/2(mot_lr) -> Mux/2
  Signals/1 -> emergency_stop/1(Signals)

== system analyze/MainControl/mode_control/forward ==
  Signals : Inport
  Action Port : ActionPort  ActionType=case
  forward : Subsystem
  forward_dem : Outport
  wires:
  forward/1(forward_dem) -> forward_dem/1
  Signals/1 -> forward/1(Signals)

== system analyze/MainControl/mode_control/neutral ==
  Signals : Inport
  Action Port : ActionPort  ActionType=case
  Mux : Mux  Inputs=6
  neutral : Subsystem
  neutral_dem : Outport
  wires:
  Mux/1 -> neutral_dem/1
  Signals/1 -> neutral/1(Signals)
  neutral/2(mot_lr) -> Mux/2
  neutral/3(mot_rf) -> Mux/3
  neutral/1(mot_lf) -> Mux/1
  neutral/6(bra_pre_r) -> Mux/6
  neutral/5(bra_pre_l) -> Mux/5
  neutral/4(mot_rr) -> Mux/4

== system analyze/OutputSignalProcess/VCU_ESC/VVMS_BrkPSetLe_MPa ==
  VVMS_BrkPSetLe_MPa : Inport
  Constant{2..8} (7 alike) : Constant  Value=0  OutDataTypeStr=uint8
  VVMS_BrkPSetLe_MPaRon : Rounding  Operator=round
  VVMS_BrkPSetLe_MPa_1sat : Saturate  UpperLimit=255  LowerLimit=0
  VVMS_BrkPSetLe_MPa_Convert : DataTypeConversion  OutDataTypeStr=uint8
  VVMS_BrkPSetLe_MPa_Convert1 : DataTypeConversion  OutDataTypeStr=uint32
  VVMS_BrkPSetLe_MPa_D : Product  Inputs=*/
  VVMS_BrkPSetLe_MPa_F : Constant  Value=0.1  OutDataTypeStr=single
  VVMS_BrkPSetLe_MPa_L : simulink/Logic and Bit Operations/Bitwise Operator  logicop=AND  UseBitMask=on  BitMask=255  BitMaskRealWorld=Stored Integer
  VVMS_BrkPSetLe_MPa_O : Constant  Value=0  OutDataTypeStr=single
  VVMS_BrkPSetLe_MPa_S : ArithShift
  VVMS_BrkPSetLe_MPa_sat : Saturate  UpperLimit=25.5  LowerLimit=0
  VVMS_BrkPSetLe_MPa_st : Sum  Inputs=+-
  output1 : Outport
  output2 : Outport  Port=2
  output3 : Outport  Port=3
  output4 : Outport  Port=4
  output5 : Outport  Port=5
  output6 : Outport  Port=6
  output7 : Outport  Port=7
  output8 : Outport  Port=8
  wires:
  VVMS_BrkPSetLe_MPa/1 -> VVMS_BrkPSetLe_MPa_sat/1
  VVMS_BrkPSetLe_MPa_sat/1 -> VVMS_BrkPSetLe_MPa_st/1
  VVMS_BrkPSetLe_MPa_O/1 -> VVMS_BrkPSetLe_MPa_st/2
  VVMS_BrkPSetLe_MPa_st/1 -> VVMS_BrkPSetLe_MPa_D/1
  VVMS_BrkPSetLe_MPa_F/1 -> VVMS_BrkPSetLe_MPa_D/2
  VVMS_BrkPSetLe_MPa_D/1 -> VVMS_BrkPSetLe_MPaRon/1
  VVMS_BrkPSetLe_MPaRon/1 -> VVMS_BrkPSetLe_MPa_S/1
  VVMS_BrkPSetLe_MPa_S/1 -> VVMS_BrkPSetLe_MPa_1sat/1
  VVMS_BrkPSetLe_MPa_1sat/1 -> VVMS_BrkPSetLe_MPa_Convert1/1
  VVMS_BrkPSetLe_MPa_Convert1/1 -> VVMS_BrkPSetLe_MPa_L/1
  VVMS_BrkPSetLe_MPa_L/1 -> VVMS_BrkPSetLe_MPa_Convert/1
  VVMS_BrkPSetLe_MPa_Convert/1 -> output1/1
  Constant2/1 -> output2/1
  Constant3/1 -> output3/1
  Constant4/1 -> output4/1
  Constant5/1 -> output5/1
  Constant6/1 -> output6/1
  Constant7/1 -> output7/1
  Constant8/1 -> output8/1

== system analyze/OutputSignalProcess/VCU_ESC/VVMS_BrkPSetRi_MPa ==
  VVMS_BrkPSetRi_MPa : Inport
  Constant{1,3..8} (7 alike) : Constant  Value=0  OutDataTypeStr=uint8
  VVMS_BrkPSetRi_MPaRon : Rounding  Operator=round
  VVMS_BrkPSetRi_MPa_1sat : Saturate  UpperLimit=255  LowerLimit=0
  VVMS_BrkPSetRi_MPa_Convert : DataTypeConversion  OutDataTypeStr=uint8
  VVMS_BrkPSetRi_MPa_Convert1 : DataTypeConversion  OutDataTypeStr=uint32
  VVMS_BrkPSetRi_MPa_D : Product  Inputs=*/
  VVMS_BrkPSetRi_MPa_F : Constant  Value=0.1  OutDataTypeStr=single
  VVMS_BrkPSetRi_MPa_L : simulink/Logic and Bit Operations/Bitwise Operator  logicop=AND  UseBitMask=on  BitMask=255  BitMaskRealWorld=Stored Integer
  VVMS_BrkPSetRi_MPa_O : Constant  Value=0  OutDataTypeStr=single
  VVMS_BrkPSetRi_MPa_S : ArithShift
  VVMS_BrkPSetRi_MPa_sat : Saturate  UpperLimit=25.5  LowerLimit=0
  VVMS_BrkPSetRi_MPa_st : Sum  Inputs=+-
  output1 : Outport
  output2 : Outport  Port=2
  output3 : Outport  Port=3
  output4 : Outport  Port=4
  output5 : Outport  Port=5
  output6 : Outport  Port=6
  output7 : Outport  Port=7
  output8 : Outport  Port=8
  wires:
  VVMS_BrkPSetRi_MPa/1 -> VVMS_BrkPSetRi_MPa_sat/1
  VVMS_BrkPSetRi_MPa_sat/1 -> VVMS_BrkPSetRi_MPa_st/1
  VVMS_BrkPSetRi_MPa_O/1 -> VVMS_BrkPSetRi_MPa_st/2
  VVMS_BrkPSetRi_MPa_st/1 -> VVMS_BrkPSetRi_MPa_D/1
  VVMS_BrkPSetRi_MPa_F/1 -> VVMS_BrkPSetRi_MPa_D/2
  VVMS_BrkPSetRi_MPa_D/1 -> VVMS_BrkPSetRi_MPaRon/1
  VVMS_BrkPSetRi_MPaRon/1 -> VVMS_BrkPSetRi_MPa_S/1
  VVMS_BrkPSetRi_MPa_S/1 -> VVMS_BrkPSetRi_MPa_1sat/1
  VVMS_BrkPSetRi_MPa_1sat/1 -> VVMS_BrkPSetRi_MPa_Convert1/1
  VVMS_BrkPSetRi_MPa_Convert1/1 -> VVMS_BrkPSetRi_MPa_L/1
  VVMS_BrkPSetRi_MPa_L/1 -> VVMS_BrkPSetRi_MPa_Convert/1
  VVMS_BrkPSetRi_MPa_Convert/1 -> output2/1
  Constant1/1 -> output1/1
  Constant3/1 -> output3/1
  Constant4/1 -> output4/1
  Constant5/1 -> output5/1
  Constant6/1 -> output6/1
  Constant7/1 -> output7/1
  Constant8/1 -> output8/1

== system analyze/OutputSignalProcess/VCU_ESC/VVMS_BrkSts_flg ==
  VVMS_BrkSts_flg : Inport
  Constant{1..2,4..8} (7 alike) : Constant  Value=0  OutDataTypeStr=uint8
  VVMS_BrkSts_flgRon : Rounding  Operator=round
  VVMS_BrkSts_flg_1sat : Saturate  UpperLimit=64  LowerLimit=0
  VVMS_BrkSts_flg_Convert : DataTypeConversion  OutDataTypeStr=uint8
  VVMS_BrkSts_flg_Convert1 : DataTypeConversion  OutDataTypeStr=uint32
  VVMS_BrkSts_flg_D : Product  Inputs=*/
  VVMS_BrkSts_flg_F : Constant  OutDataTypeStr=single
  VVMS_BrkSts_flg_L : simulink/Logic and Bit Operations/Bitwise Operator  logicop=AND  UseBitMask=on  BitMask=64  BitMaskRealWorld=Stored Integer
  VVMS_BrkSts_flg_O : Constant  Value=0  OutDataTypeStr=single
  VVMS_BrkSts_flg_S : ArithShift  BitShiftNumber=-6
  VVMS_BrkSts_flg_sat : Saturate  UpperLimit=1  LowerLimit=0
  VVMS_BrkSts_flg_st : Sum  Inputs=+-
  output1 : Outport
  output2 : Outport  Port=2
  output3 : Outport  Port=3
  output4 : Outport  Port=4
  output5 : Outport  Port=5
  output6 : Outport  Port=6
  output7 : Outport  Port=7
  output8 : Outport  Port=8
  wires:
  VVMS_BrkSts_flg/1 -> VVMS_BrkSts_flg_sat/1
  VVMS_BrkSts_flg_sat/1 -> VVMS_BrkSts_flg_st/1
  VVMS_BrkSts_flg_O/1 -> VVMS_BrkSts_flg_st/2
  VVMS_BrkSts_flg_st/1 -> VVMS_BrkSts_flg_D/1
  VVMS_BrkSts_flg_F/1 -> VVMS_BrkSts_flg_D/2
  VVMS_BrkSts_flg_D/1 -> VVMS_BrkSts_flgRon/1
  VVMS_BrkSts_flgRon/1 -> VVMS_BrkSts_flg_S/1
  VVMS_BrkSts_flg_S/1 -> VVMS_BrkSts_flg_1sat/1
  VVMS_BrkSts_flg_1sat/1 -> VVMS_BrkSts_flg_Convert1/1
  VVMS_BrkSts_flg_Convert1/1 -> VVMS_BrkSts_flg_L/1
  VVMS_BrkSts_flg_L/1 -> VVMS_BrkSts_flg_Convert/1
  VVMS_BrkSts_flg_Convert/1 -> output3/1
  Constant1/1 -> output1/1
  Constant2/1 -> output2/1
  Constant4/1 -> output4/1
  Constant5/1 -> output5/1
  Constant6/1 -> output6/1
  Constant7/1 -> output7/1
  Constant8/1 -> output8/1
